simulink model "problem16"  (R2021a)
settings: Solver=VariableStepAuto  StartTime=0.0  StopTime=10.0  RelTol=1e-3
undefined symbols (not defined in the file): B, J1, J2, J3, J4, Kd_1, Kd_2, Kd_3, Kd_4, Ki_1, Ki_2, Ki_3, Ki_4, Kp_1, Kp_2, Kp_3, Kp_4, n, qr_1, qr_2, qr_3, qr_4, T1, T2, T3, T4
settings Model: Creator=Luky  LastModifiedBy=Luky

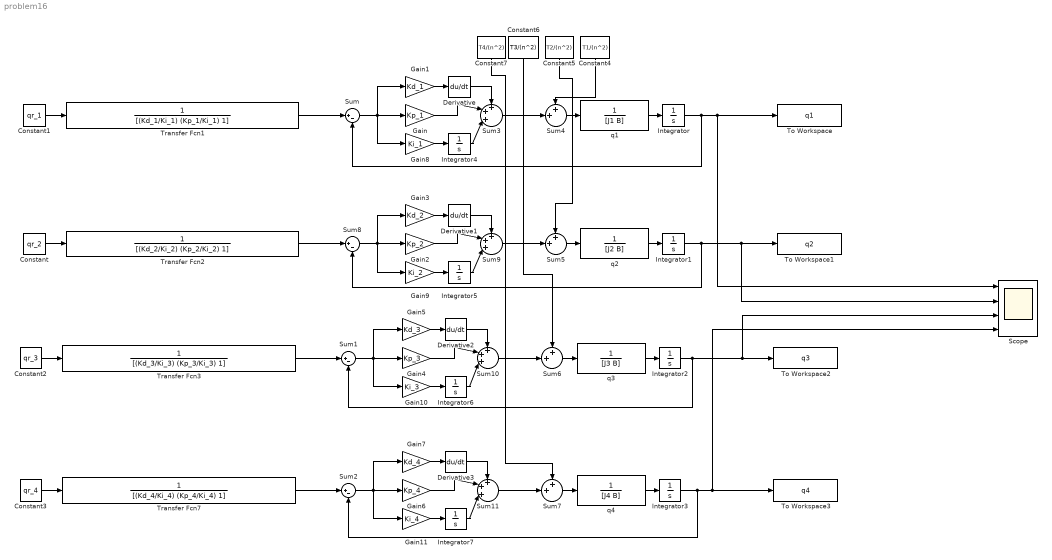
== system problem16 ==
  Constant : Constant  Value=qr_2
  Constant1 : Constant  Value=qr_1
  Constant2 : Constant  Value=qr_3
  Constant3 : Constant  Value=qr_4
  Constant4 : Constant  Value=T1/(n^2)
  Constant5 : Constant  Value=T2/(n^2)
  Constant6 : Constant  Value=T3/(n^2)
  Constant7 : Constant  Value=T4/(n^2)
  Derivative{,1..3} (4 alike) : Derivative
  Gain : Gain  Gain=Kp_1
  Gain1 : Gain  Gain=Kd_1
  Gain10 : Gain  Gain=Ki_3
  Gain11 : Gain  Gain=Ki_4
  Gain2 : Gain  Gain=Kp_2
  Gain3 : Gain  Gain=Kd_2
  Gain4 : Gain  Gain=Kp_3
  Gain5 : Gain  Gain=Kd_3
  Gain6 : Gain  Gain=Kp_4
  Gain7 : Gain  Gain=Kd_4
  Gain8 : Gain  Gain=Ki_1
  Gain9 : Gain  Gain=Ki_2
  Integrator{,1..7} (8 alike) : Integrator
  Scope : Scope  NumInputPorts=4
  Sum{,1..2,8} (4 alike) : Sum  Inputs=|+-
  Sum{3,9..11} (4 alike) : Sum  Inputs=+++|
  Sum{4..7} (4 alike) : Sum  Inputs=++|
  To Workspace : ToWorkspace  VariableName=q1  SaveFormat=Timeseries  SampleTime=-1
  To Workspace1 : ToWorkspace  VariableName=q2  SaveFormat=Timeseries  SampleTime=-1
  To Workspace2 : ToWorkspace  VariableName=q3  SaveFormat=Timeseries  SampleTime=-1
  To Workspace3 : ToWorkspace  VariableName=q4  SaveFormat=Timeseries  SampleTime=-1
  Transfer Fcn1 : TransferFcn  Denominator=[(Kd_1/Ki_1) (Kp_1/Ki_1) 1]
  Transfer Fcn2 : TransferFcn  Denominator=[(Kd_2/Ki_2) (Kp_2/Ki_2) 1]
  Transfer Fcn3 : TransferFcn  Denominator=[(Kd_3/Ki_3) (Kp_3/Ki_3) 1]
  Transfer Fcn7 : TransferFcn  Denominator=[(Kd_4/Ki_4) (Kp_4/Ki_4) 1]
  q1 : TransferFcn  Denominator=[J1 B]
  q2 : TransferFcn  Denominator=[J2 B]
  q3 : TransferFcn  Denominator=[J3 B]
  q4 : TransferFcn  Denominator=[J4 B]
  wires:
  Constant1/1 -> Transfer Fcn1/1
  Constant/1 -> Transfer Fcn2/1
  Constant2/1 -> Transfer Fcn3/1
  Constant3/1 -> Transfer Fcn7/1
  Gain5/1 -> Derivative2/1
  Sum/1 -> Gain8/1, Gain1/1, Gain/1
  Derivative3/1 -> Sum11/1
  Integrator6/1 -> Sum10/3
  Gain10/1 -> Integrator6/1
  Integrator7/1 -> Sum11/3
  Gain11/1 -> Integrator7/1
  Transfer Fcn1/1 -> Sum/1
  Gain/1 -> Sum3/2
  Gain4/1 -> Sum10/2
  Transfer Fcn7/1 -> Sum2/1
  Sum11/1 -> Sum7/2
  Gain2/1 -> Sum9/2
  Integrator5/1 -> Sum9/3
  Sum10/1 -> Sum6/2
  Gain8/1 -> Integrator4/1
  Sum4/1 -> q1/1
  Gain7/1 -> Derivative3/1
  Integrator4/1 -> Sum3/3
  Gain6/1 -> Sum11/2
  Gain3/1 -> Derivative1/1
  Derivative2/1 -> Sum10/1
  Sum8/1 -> Gain9/1, Gain3/1, Gain2/1
  Integrator3/1 -> Sum2/2, Scope/4, To Workspace3/1
  Derivative/1 -> Sum3/1
  Sum1/1 -> Gain10/1, Gain5/1, Gain4/1
  Integrator1/1 -> Sum8/2, Scope/2, To Workspace1/1
  Gain9/1 -> Integrator5/1
  Sum9/1 -> Sum5/2
  Gain1/1 -> Derivative/1
  Derivative1/1 -> Sum9/1
  Sum6/1 -> q3/1
  Integrator2/1 -> Sum1/2, Scope/3, To Workspace2/1
  Transfer Fcn3/1 -> Sum1/1
  Sum2/1 -> Gain11/1, Gain7/1, Gain6/1
  Transfer Fcn2/1 -> Sum8/1
  Sum3/1 -> Sum4/2
  Sum7/1 -> q4/1
  q4/1 -> Integrator3/1
  q2/1 -> Integrator1/1
  Integrator/1 -> Sum/2, Scope/1, To Workspace/1
  Sum5/1 -> q2/1
  q3/1 -> Integrator2/1
  q1/1 -> Integrator/1
  Constant6/1 -> Sum6/1
  Constant7/1 -> Sum7/1
  Constant5/1 -> Sum5/1
  Constant4/1 -> Sum4/1
